simulink model "Final_Leg_PurePursuit_Squat_Climb"  (R2025b)
settings: Solver=ode45  StartTime=0.0  StopTime=150  MaxStep=0.002  RelTol=0.01  AbsTol=0.01  EnableMultiTasking=on
undefined symbols (not defined in the file): waypoints, X, Y, Z
libraries: sm_lib x81, nesl_utility x35, slpidlib x2, robotalgslib x1, sharedtransform x1
(part 4 of 5)

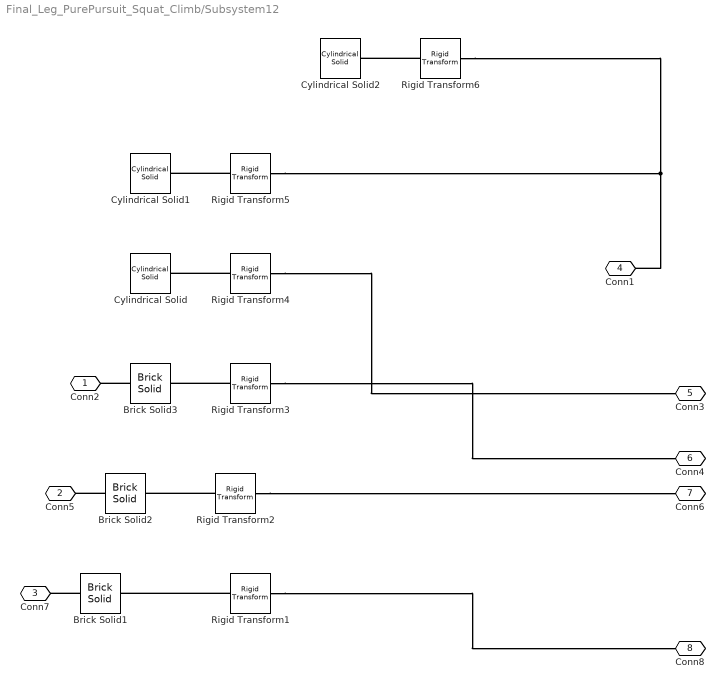
== system Final_Leg_PurePursuit_Squat_Climb/Subsystem12 ==
  Brick Solid1 : sm_lib/Body Elements/Brick Solid  BrickDimensions=[14.5 7.3 2]  BrickDimensionsUnits=m  ExportEntireGeometry=on  InertiaType=CalculateFromGeometry  BasedOnType=Density  Density=1000  DensityUnits=kg/m^3  Mass=1  MassUnits=kg  CenterOfMass=[0 0 0]  CenterOfMassUnits=m  MomentsOfInertia=[1 1 1]  MomentsOfInertiaUnits=kg*m^2  ProductsOfInertia=[0 0 0]  ProductsOfInertiaUnits=kg*m^2  GraphicType=FromGeometry  MarkerShape=Sphere  MarkerSize=10  GraphicVisPropType=SimpleVisualProperties  GraphicDiffuseColor=[0.3333 0.1882 0.007843]  GraphicOpacity=1  GraphicSpecularColor=[0.5 0.5 0.5 1.0]  GraphicAmbientColor=[0.15 0.15 0.15 1.0]  GraphicEmissiveColor=[0.0 0.0 0.0 1.0]  GraphicShininess=75  DoExposeReferenceFrame=on  SerializedFrames=<Frames/>
  Brick Solid2 : sm_lib/Body Elements/Brick Solid  BrickDimensions=[12.4 9.9 2]  BrickDimensionsUnits=m  ExportEntireGeometry=on  InertiaType=CalculateFromGeometry  BasedOnType=Density  Density=1000  DensityUnits=kg/m^3  Mass=1  MassUnits=kg  CenterOfMass=[0 0 0]  CenterOfMassUnits=m  MomentsOfInertia=[1 1 1]  MomentsOfInertiaUnits=kg*m^2  ProductsOfInertia=[0 0 0]  ProductsOfInertiaUnits=kg*m^2  GraphicType=FromGeometry  MarkerShape=Sphere  MarkerSize=10  GraphicVisPropType=SimpleVisualProperties  GraphicDiffuseColor=[0.3333 0.1882 0.007843]  GraphicOpacity=1  GraphicSpecularColor=[0.5 0.5 0.5 1.0]  GraphicAmbientColor=[0.15 0.15 0.15 1.0]  GraphicEmissiveColor=[0.0 0.0 0.0 1.0]  GraphicShininess=75  DoExposeReferenceFrame=on  SerializedFrames=<Frames/>
  Brick Solid3 : sm_lib/Body Elements/Brick Solid  BrickDimensions=[10 10 2]  BrickDimensionsUnits=m  ExportEntireGeometry=on  InertiaType=CalculateFromGeometry  BasedOnType=Density  Density=1000  DensityUnits=kg/m^3  Mass=1  MassUnits=kg  CenterOfMass=[0 0 0]  CenterOfMassUnits=m  MomentsOfInertia=[1 1 1]  MomentsOfInertiaUnits=kg*m^2  ProductsOfInertia=[0 0 0]  ProductsOfInertiaUnits=kg*m^2  GraphicType=FromGeometry  MarkerShape=Sphere  MarkerSize=10  GraphicVisPropType=SimpleVisualProperties  GraphicDiffuseColor=[0.3333 0.1882 0.007843]  GraphicOpacity=1  GraphicSpecularColor=[0.5 0.5 0.5 1.0]  GraphicAmbientColor=[0.15 0.15 0.15 1.0]  GraphicEmissiveColor=[0.0 0.0 0.0 1.0]  GraphicShininess=75  DoExposeReferenceFrame=on  SerializedFrames=<Frames/>
  Cylindrical Solid : sm_lib/Body Elements/Cylindrical Solid  CylinderRadius=6  CylinderRadiusUnits=m  CylinderLength=2  CylinderLengthUnits=m  ExportEntireGeometry=off  InertiaType=CalculateFromGeometry  BasedOnType=Density  Density=1000  DensityUnits=kg/m^3  Mass=1  MassUnits=kg  CenterOfMass=[0 0 0]  CenterOfMassUnits=m  MomentsOfInertia=[1 1 1]  MomentsOfInertiaUnits=kg*m^2  ProductsOfInertia=[0 0 0]  ProductsOfInertiaUnits=kg*m^2  GraphicType=FromGeometry  MarkerShape=Sphere  MarkerSize=10  GraphicVisPropType=SimpleVisualProperties  GraphicDiffuseColor=[0.3333 0.1882 0.007843]  GraphicOpacity=1  GraphicSpecularColor=[0.5 0.5 0.5 1.0]  GraphicAmbientColor=[0.15 0.15 0.15 1.0]  GraphicEmissiveColor=[0.0 0.0 0.0 1.0]  GraphicShininess=75  DoExposeReferenceFrame=on  SerializedFrames=<Frames/>
  Cylindrical Solid1 : sm_lib/Body Elements/Cylindrical Solid  CylinderRadius=5  CylinderRadiusUnits=m  CylinderLength=2  CylinderLengthUnits=m  ExportEntireGeometry=off  InertiaType=CalculateFromGeometry  BasedOnType=Density  Density=1000  DensityUnits=kg/m^3  Mass=1  MassUnits=kg  CenterOfMass=[0 0 0]  CenterOfMassUnits=m  MomentsOfInertia=[1 1 1]  MomentsOfInertiaUnits=kg*m^2  ProductsOfInertia=[0 0 0]  ProductsOfInertiaUnits=kg*m^2  GraphicType=FromGeometry  MarkerShape=Sphere  MarkerSize=10  GraphicVisPropType=SimpleVisualProperties  GraphicDiffuseColor=[0.3333 0.1882 0.007843]  GraphicOpacity=1  GraphicSpecularColor=[0.5 0.5 0.5 1.0]  GraphicAmbientColor=[0.15 0.15 0.15 1.0]  GraphicEmissiveColor=[0.0 0.0 0.0 1.0]  GraphicShininess=75  DoExposeReferenceFrame=on  SerializedFrames=<Frames/>
  Cylindrical Solid2 : sm_lib/Body Elements/Cylindrical Solid  CylinderRadius=5  CylinderRadiusUnits=m  CylinderLength=2  CylinderLengthUnits=m  ExportEntireGeometry=off  InertiaType=CalculateFromGeometry  BasedOnType=Density  Density=1000  DensityUnits=kg/m^3  Mass=1  MassUnits=kg  CenterOfMass=[0 0 0]  CenterOfMassUnits=m  MomentsOfInertia=[1 1 1]  MomentsOfInertiaUnits=kg*m^2  ProductsOfInertia=[0 0 0]  ProductsOfInertiaUnits=kg*m^2  GraphicType=FromGeometry  MarkerShape=Sphere  MarkerSize=10  GraphicVisPropType=SimpleVisualProperties  GraphicDiffuseColor=[0.3333 0.1882 0.007843]  GraphicOpacity=1  GraphicSpecularColor=[0.5 0.5 0.5 1.0]  GraphicAmbientColor=[0.15 0.15 0.15 1.0]  GraphicEmissiveColor=[0.0 0.0 0.0 1.0]  GraphicShininess=75  DoExposeReferenceFrame=on  SerializedFrames=<Frames/>
  Rigid Transform1 : sm_lib/Frames and Transforms/Rigid Transform  RotationMethod=None  FollAlignAxisA=+X  BaseAlignAxisA=+Y  FollAlignAxisB=+Y  BaseAlignAxisB=+Z  RotationStandardAxis=+Z  RotationAngle=90  RotationAngleUnits=deg  RotationArbitraryAxis=[0 0 1]  RotationSequenceAxes=FollowerAxes  RotationSequence=XYX  RotationSequenceAngles=[0 0 0]  RotationSequenceAnglesUnits=deg  RotationMatrix=[1 0 0;0 1 0;0 0 1]  Quaternion=[1 0 0 0]  TranslationMethod=Cartesian  TranslationCartesianOffset=[-15 -13.75 -1]  TranslationCartesianOffsetUnits=m  TranslationStandardAxis=+Z  TranslationStandardOffset=0  TranslationStandardOffsetUnits=m  TranslationROffset=0  TranslationROffsetUnits=m  TranslationThetaOffset=0  TranslationThetaOffsetUnits=deg  TranslationZOffset=0  TranslationZOffsetUnits=m
  Rigid Transform2 : sm_lib/Frames and Transforms/Rigid Transform  RotationMethod=None  FollAlignAxisA=+X  BaseAlignAxisA=+Y  FollAlignAxisB=+Y  BaseAlignAxisB=+Z  RotationStandardAxis=+Z  RotationAngle=90  RotationAngleUnits=deg  RotationArbitraryAxis=[0 0 1]  RotationSequenceAxes=FollowerAxes  RotationSequence=XYX  RotationSequenceAngles=[0 0 0]  RotationSequenceAnglesUnits=deg  RotationMatrix=[1 0 0;0 1 0;0 0 1]  Quaternion=[1 0 0 0]  TranslationMethod=Cartesian  TranslationCartesianOffset=[-21 -32.5 -1]  TranslationCartesianOffsetUnits=m  TranslationStandardAxis=+Z  TranslationStandardOffset=0  TranslationStandardOffsetUnits=m  TranslationROffset=0  TranslationROffsetUnits=m  TranslationThetaOffset=0  TranslationThetaOffsetUnits=deg  TranslationZOffset=0  TranslationZOffsetUnits=m
  Rigid Transform3 : sm_lib/Frames and Transforms/Rigid Transform  RotationMethod=None  FollAlignAxisA=+X  BaseAlignAxisA=+Y  FollAlignAxisB=+Y  BaseAlignAxisB=+Z  RotationStandardAxis=+Z  RotationAngle=90  RotationAngleUnits=deg  RotationArbitraryAxis=[0 0 1]  RotationSequenceAxes=FollowerAxes  RotationSequence=XYX  RotationSequenceAngles=[0 0 0]  RotationSequenceAnglesUnits=deg  RotationMatrix=[1 0 0;0 1 0;0 0 1]  Quaternion=[1 0 0 0]  TranslationMethod=Cartesian  TranslationCartesianOffset=[-37.5 -15 -1]  TranslationCartesianOffsetUnits=m  TranslationStandardAxis=+Z  TranslationStandardOffset=0  TranslationStandardOffsetUnits=m  TranslationROffset=0  TranslationROffsetUnits=m  TranslationThetaOffset=0  TranslationThetaOffsetUnits=deg  TranslationZOffset=0  TranslationZOffsetUnits=m
  Rigid Transform4 : sm_lib/Frames and Transforms/Rigid Transform  RotationMethod=None  FollAlignAxisA=+X  BaseAlignAxisA=+Y  FollAlignAxisB=+Y  BaseAlignAxisB=+Z  RotationStandardAxis=+Z  RotationAngle=90  RotationAngleUnits=deg  RotationArbitraryAxis=[0 0 1]  RotationSequenceAxes=FollowerAxes  RotationSequence=XYX  RotationSequenceAngles=[0 0 0]  RotationSequenceAnglesUnits=deg  RotationMatrix=[1 0 0;0 1 0;0 0 1]  Quaternion=[1 0 0 0]  TranslationMethod=Cartesian  TranslationCartesianOffset=[-15 -37.5 -1]  TranslationCartesianOffsetUnits=m  TranslationStandardAxis=+Z  TranslationStandardOffset=0  TranslationStandardOffsetUnits=m  TranslationROffset=0  TranslationROffsetUnits=m  TranslationThetaOffset=0  TranslationThetaOffsetUnits=deg  TranslationZOffset=0  TranslationZOffsetUnits=m
  Rigid Transform5 : sm_lib/Frames and Transforms/Rigid Transform  RotationMethod=None  FollAlignAxisA=+X  BaseAlignAxisA=+Y  FollAlignAxisB=+Y  BaseAlignAxisB=+Z  RotationStandardAxis=+Z  RotationAngle=90  RotationAngleUnits=deg  RotationArbitraryAxis=[0 0 1]  RotationSequenceAxes=FollowerAxes  RotationSequence=XYX  RotationSequenceAngles=[0 0 0]  RotationSequenceAnglesUnits=deg  RotationMatrix=[1 0 0;0 1 0;0 0 1]  Quaternion=[1 0 0 0]  TranslationMethod=Cartesian  TranslationCartesianOffset=[-35 -30 -1]  TranslationCartesianOffsetUnits=m  TranslationStandardAxis=+Z  TranslationStandardOffset=0  TranslationStandardOffsetUnits=m  TranslationROffset=0  TranslationROffsetUnits=m  TranslationThetaOffset=0  TranslationThetaOffsetUnits=deg  TranslationZOffset=0  TranslationZOffsetUnits=m
  Rigid Transform6 : sm_lib/Frames and Transforms/Rigid Transform  RotationMethod=None  FollAlignAxisA=+X  BaseAlignAxisA=+Y  FollAlignAxisB=+Y  BaseAlignAxisB=+Z  RotationStandardAxis=+Z  RotationAngle=90  RotationAngleUnits=deg  RotationArbitraryAxis=[0 0 1]  RotationSequenceAxes=FollowerAxes  RotationSequence=XYX  RotationSequenceAngles=[0 0 0]  RotationSequenceAnglesUnits=deg  RotationMatrix=[1 0 0;0 1 0;0 0 1]  Quaternion=[1 0 0 0]  TranslationMethod=Cartesian  TranslationCartesianOffset=[-25 -12.5 -1]  TranslationCartesianOffsetUnits=m  TranslationStandardAxis=+Z  TranslationStandardOffset=0  TranslationStandardOffsetUnits=m  TranslationROffset=0  TranslationROffsetUnits=m  TranslationThetaOffset=0  TranslationThetaOffsetUnits=deg  TranslationZOffset=0  TranslationZOffsetUnits=m
  Conn2 : PMIOPort  Side=Left
  Conn5 : PMIOPort  Port=2  Side=Left
  Conn7 : PMIOPort  Port=3  Side=Left
  Conn1 : PMIOPort  Port=4  Side=Right
  Conn3 : PMIOPort  Port=5  Side=Right
  Conn4 : PMIOPort  Port=6  Side=Right
  Conn6 : PMIOPort  Port=7  Side=Right
  Conn8 : PMIOPort  Port=8  Side=Right
  connections:
  Rigid Transform1/LConn1 -- Brick Solid1/RConn1
  Rigid Transform5/LConn1 -- Cylindrical Solid1/RConn1
  Rigid Transform3/LConn1 -- Brick Solid3/RConn1
  Rigid Transform5/RConn1 -- Conn1/RConn1 -- Rigid Transform6/RConn1
  Brick Solid2/LConn1 -- Conn5/RConn1
  Rigid Transform1/RConn1 -- Conn8/RConn1
  Rigid Transform4/RConn1 -- Conn3/RConn1
  Rigid Transform6/LConn1 -- Cylindrical Solid2/RConn1
  Rigid Transform4/LConn1 -- Cylindrical Solid/RConn1
  Rigid Transform2/LConn1 -- Brick Solid2/RConn1
  Rigid Transform3/RConn1 -- Conn4/RConn1
  Rigid Transform2/RConn1 -- Conn6/RConn1
  Brick Solid1/LConn1 -- Conn7/RConn1
  Brick Solid3/LConn1 -- Conn2/RConn1

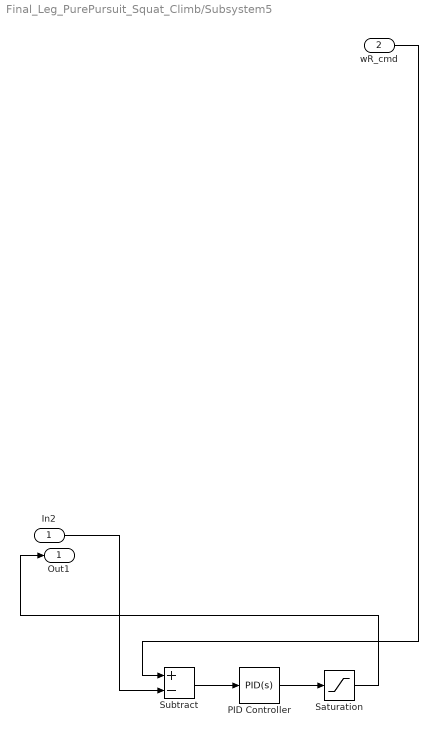
== system Final_Leg_PurePursuit_Squat_Climb/Subsystem5 ==
  In2 : Inport
  wR_cmd : Inport  Port=2
  PID Controller : slpidlib/PID Controller  Controller=PID  Form=Parallel  TimeDomain=Continuous-time  UseExternalTs=off  SampleTime=-1  IntegratorMethod=Forward Euler  FilterMethod=Forward Euler  ControllerParametersSource=internal  P=5  I=0  UseKiTs=off  D=0  UseExternalDerivativeSource=off  N=100  UseFilter=on  TunerSelectOption=Transfer Function Based (PID Tuner App)  InitialConditionSource=internal  InitialConditionForIntegrator=0  InitialConditionForFilter=0  DifferentiatorICPrevScaledInput=0  ExternalReset=none  TrackingMode=off  Kt=1  LimitOutput=off  SatLimitsSource=internal  UpperSaturationLimit=inf  LowerSaturationLimit=-inf  LinearizeAsGain=on  AntiWindupMode=none  Kb=1  LimitIntegrator=off  UpperIntegratorSaturationLimit=inf  LowerIntegratorSaturationLimit=-inf  POutMin=[]  POutMax=[]  IOutMin=[]  IOutMax=[]  DOutMin=[]  DOutMax=[]  NOutMin=[]  NOutMax=[]  SumOutMin=[]  SumOutMax=[]  SaturationOutMin=[]  SaturationOutMax=[]  PParamMin=[]  PParamMax=[]  IParamMin=[]  IParamMax=[]  DParamMin=[]  DParamMax=[]  NParamMin=[]  NParamMax=[]  KbParamMin=[]  KbParamMax=[]  KtParamMin=[]  KtParamMax=[]  KbOutMin=[]  KbOutMax=[]  KtOutMin=[]  KtOutMax=[]  IntegratorOutMin=[]  IntegratorOutMax=[]  FilterOutMin=[]  FilterOutMax=[]  SumI1OutMin=[]  SumI1OutMax=[]  SumI2OutMin=[]  SumI2OutMax=[]  SumI3OutMin=[]  SumI3OutMax=[]  SumI4OutMin=[]  SumI4OutMax=[]  SumDOutMin=[]  SumDOutMax=[]  DifferentiatorOutMin=[]  DifferentiatorOutMax=[]  FilterDiffOutCoefMin=[]  FilterDiffOutCoefMax=[]  ReciprocalOutMin=[]  ReciprocalOutMax=[]  SumDenOutMin=[]  SumDenOutMax=[]  SumNumOutMin=[]  SumNumOutMax=[]  DivideOutMin=[]  DivideOutMax=[]  UdiffTsProdOutMin=[]  UdiffTsProdOutMax=[]  NTsProdOutMin=[]  NTsProdOutMax=[]  UintegralTsProdOutMin=[]  UintegralTsProdOutMax=[]  UngainTsProdOutMin=[]  UngainTsProdOutMax=[]  ClampingZeroOutDataTypeStr=Inherit: Inherit via back propagation  ClampingZeroOutMin=[]  ClampingZeroOutMax=[]  FilterDenConstantOutDataTypeStr=Inherit: Inherit via back propagation  FilterDenConstantOutMin=[]  FilterDenConstantOutMax=[]  PCopyOutDataTypeStr=Inherit: Inherit via back propagation  PCopyOutMin=[]  PCopyOutMax=[]  NCopyOutDataTypeStr=Inherit: Inherit via back propagation  NCopyOutMin=[]  NCopyOutMax=[]  IntegratorContinuousStateAttributes=''  IntegratorStateMustResolveToSignalObject=off  IntegratorRTWStateStorageClass=Auto  FilterContinuousStateAttributes=''  FilterStateMustResolveToSignalObject=off  FilterRTWStateStorageClass=Auto  ParallelPVariant=InternalParameters  IdealPVariant=Disabled  IVariant=InternalParameters  DVariant=InternalParameters  IntegratorVariant=Continuous  SatVariant=Disabled  AWVariant=Passthrough  PCopyVariant=Disabled  TRVariant=Disabled  FdbkBlocksVariant=Forward  IdealPFdbkVariant=Disabled  SatFdbkVariant=Disabled  DerivativeFilterVariant=ContFilter  NVariant=InternalParameters  NCopyVariant=Disabled  FilterICVariant=InternalICsFilter  IntegratorICVariant=InternalICs  ExternalResetVariant=Disabled  TRSumVariant=Passthrough  SumFdbkVariant=Disabled  SumVariant=Sum_PID  TsampFilterVariant=InternalTs  TsampNgainVariant=Passthrough  TsampIntegralVariant=Disabled_SignalSpec  ExternalSaturationOutDataTypeStr=Inherit: Same as second input  DerivativeSourceVariant=ErrorSignal  PreIntVariant=InternalPreInt
  Saturation : Saturate  UpperLimit=5  LowerLimit=-5
  Subtract : Sum  Inputs=+-
  Out1 : Outport
  wires:
  In2/1 -> Subtract/2
  Subtract/1 -> PID Controller/1
  Saturation/1 -> Out1/1
  PID Controller/1 -> Saturation/1
  wR_cmd/1 -> Subtract/1

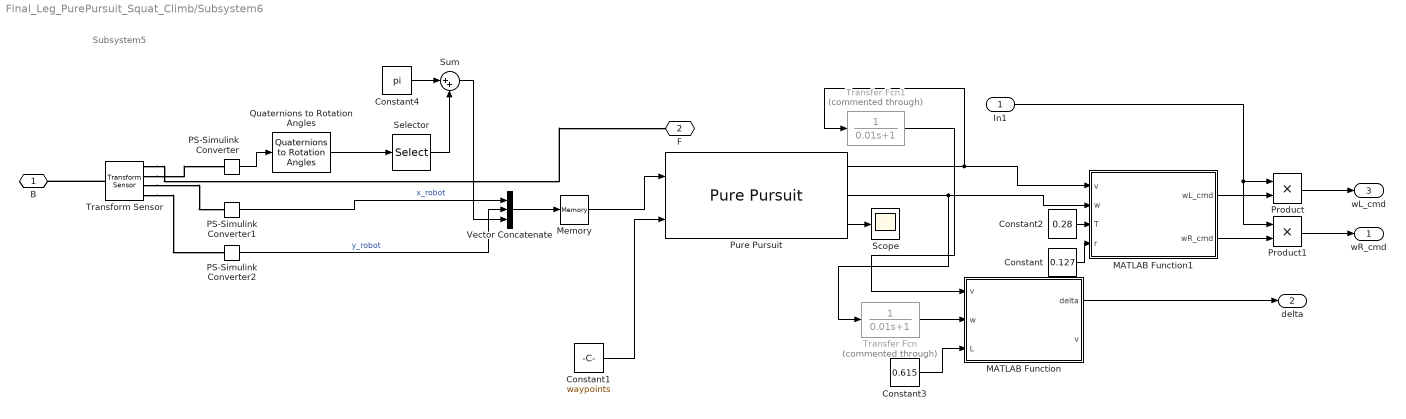
== system Final_Leg_PurePursuit_Squat_Climb/Subsystem6 ==
  note: Subsystem5
  In1 : Inport
  Constant : Constant  Value=0.127
  Constant1 : Constant  Value=waypoints
  Constant2 : Constant  Value=0.28
  Constant3 : Constant  Value=0.615
  Constant4 : Constant  Value=pi
  MATLAB Function : MATLAB Function  TreatAsAtomicUnit=on
  MATLAB Function1 : MATLAB Function  TreatAsAtomicUnit=on
  Memory : Memory
  PS-Simulink Converter : nesl_utility/PS-Simulink Converter  PhysicalDomain=network_engine_domain  SubClassName=ps_output  LeftPortType=input  RightPortType=output  PseudoPeriodic=off  Frequencies=[]  VectorFormat=inherit  Unit=inherit  AffineConversion=off
  PS-Simulink Converter1 : nesl_utility/PS-Simulink Converter  PhysicalDomain=network_engine_domain  SubClassName=ps_output  LeftPortType=input  RightPortType=output  PseudoPeriodic=off  Frequencies=[]  VectorFormat=inherit  Unit=inherit  AffineConversion=off
  PS-Simulink Converter2 : nesl_utility/PS-Simulink Converter  PhysicalDomain=network_engine_domain  SubClassName=ps_output  LeftPortType=input  RightPortType=output  PseudoPeriodic=off  Frequencies=[]  VectorFormat=inherit  Unit=inherit  AffineConversion=off
  Product : Product
  Product1 : Product
  Pure Pursuit : robotalgslib/Pure Pursuit  DesiredLinearVelocityPort=off  DesiredLinearVelocity=0.7  MaxAngularVelocity=0.8  LookaheadDistancePort=off  LookaheadDistance=0.6  TargetDirPort=on  SimulateUsing=Code generation
      settings: LibrarySourceBlock=navlib/Control Algorithms/Pure Pursuit
  Quaternions to Rotation Angles : sharedtransform/Quaternions to Rotation Angles  rotationOrder=ZYX  aMode=aMode
  Scope : Scope
      settings: ActiveDisplayYMinimum=-49.938512022124293  ActiveDisplayYMaximum=229.50278461957694
  Selector : Selector  InputPortWidth=3  IndexOptions=Index vector (dialog)  Indices=[1]  OutputSizes=1
  Sum : Sum  Inputs=|++
  Transfer Fcn : TransferFcn  Commented=through  Denominator=[0.01 1]
  Transfer Fcn1 : TransferFcn  Commented=through  Denominator=[0.01 1]
  Transform Sensor : sm_lib/Frames and Transforms/Transform Sensor  MeasurementFrame=World  RotationSequence=XYX  SenseAngle=off  SenseAxis=off  SenseQ=on  SenseR=off  SenseRotationSequence=off  SenseOmegaX=off  SenseOmegaY=off  SenseOmegaZ=off  SenseOmega=off  SenseQDot=off  SenseRDot=off  SenseRotationSequenceDot=off  SenseAlphaX=off  SenseAlphaY=off  SenseAlphaZ=off  SenseAlpha=off  SenseQDDot=off  SenseRDDot=off  SenseX=on  SenseY=on  SenseZ=off  SenseXYZ=off  SenseRad=off  SenseAzim=off  SenseDist=off  SenseInc=off  SenseXDot=off  SenseYDot=off  SenseZDot=off  SenseXYZDot=off  SenseRadDot=off  SenseAzimDot=off  SenseDistDot=off  SenseIncDot=off  SenseXDDot=off  SenseYDDot=off  SenseZDDot=off  SenseXYZDDot=off  SenseRadDDot=off  SenseAzimDDot=off  SenseDistDDot=off  SenseIncDDot=off
  Vector Concatenate : Concatenate  NumInputs=3
  B : PMIOPort  Side=Right
  F : PMIOPort  Port=2  Side=Right
  wR_cmd : Outport
  delta : Outport  Port=2
  wL_cmd : Outport  Port=3
  wires:
  Pure Pursuit/2 -> MATLAB Function1/2(w), Transfer Fcn/1
  Transfer Fcn1/1 -> MATLAB Function/1("v ")
  Transfer Fcn/1 -> MATLAB Function/2(w)
  Constant1/1 -> Pure Pursuit/2
  Constant/1 -> MATLAB Function1/4(r)
  Constant2/1 -> MATLAB Function1/3(T)
  Constant3/1 -> MATLAB Function/3(L)
  Pure Pursuit/1 -> MATLAB Function1/1(v), Transfer Fcn1/1
  Pure Pursuit/3 -> Scope/1
  Memory/1 -> Pure Pursuit/1
  In1/1 -> Product/1, Product1/1
  MATLAB Function1/1(wL_cmd) -> Product/2
  Product/1 -> wL_cmd/1
  MATLAB Function1/2(wR_cmd) -> Product1/2
  Product1/1 -> wR_cmd/1
  MATLAB Function/1(delta) -> delta/1
  Sum/1 -> Vector Concatenate/3
  Selector/1 -> Sum/2
  Constant4/1 -> Sum/1
  PS-Simulink Converter2/1 -> Vector Concatenate/2  "y_robot"
  PS-Simulink Converter1/1 -> Vector Concatenate/1  "x_robot"
  Vector Concatenate/1 -> Memory/1
  PS-Simulink Converter/1 -> Quaternions to Rotation Angles/1
  Quaternions to Rotation Angles/1 -> Selector/1
  connections:
  Transform Sensor/RConn1 -- F/RConn1
  Transform Sensor/LConn1 -- B/RConn1
  Transform Sensor/RConn3 -- PS-Simulink Converter1/LConn1
  Transform Sensor/RConn2 -- PS-Simulink Converter/LConn1
  Transform Sensor/RConn4 -- PS-Simulink Converter2/LConn1

== system Final_Leg_PurePursuit_Squat_Climb/Subsystem7 ==
  wL_cmd : Inport
  In2 : Inport  Port=2
  PID Controller : slpidlib/PID Controller  Controller=PID  Form=Parallel  TimeDomain=Continuous-time  UseExternalTs=off  SampleTime=-1  IntegratorMethod=Forward Euler  FilterMethod=Forward Euler  ControllerParametersSource=internal  P=5  I=0  UseKiTs=off  D=0  UseExternalDerivativeSource=off  N=100  UseFilter=on  TunerSelectOption=Transfer Function Based (PID Tuner App)  InitialConditionSource=internal  InitialConditionForIntegrator=0  InitialConditionForFilter=0  DifferentiatorICPrevScaledInput=0  ExternalReset=none  TrackingMode=off  Kt=1  LimitOutput=off  SatLimitsSource=internal  UpperSaturationLimit=inf  LowerSaturationLimit=-inf  LinearizeAsGain=on  AntiWindupMode=none  Kb=1  LimitIntegrator=off  UpperIntegratorSaturationLimit=inf  LowerIntegratorSaturationLimit=-inf  POutMin=[]  POutMax=[]  IOutMin=[]  IOutMax=[]  DOutMin=[]  DOutMax=[]  NOutMin=[]  NOutMax=[]  SumOutMin=[]  SumOutMax=[]  SaturationOutMin=[]  SaturationOutMax=[]  PParamMin=[]  PParamMax=[]  IParamMin=[]  IParamMax=[]  DParamMin=[]  DParamMax=[]  NParamMin=[]  NParamMax=[]  KbParamMin=[]  KbParamMax=[]  KtParamMin=[]  KtParamMax=[]  KbOutMin=[]  KbOutMax=[]  KtOutMin=[]  KtOutMax=[]  IntegratorOutMin=[]  IntegratorOutMax=[]  FilterOutMin=[]  FilterOutMax=[]  SumI1OutMin=[]  SumI1OutMax=[]  SumI2OutMin=[]  SumI2OutMax=[]  SumI3OutMin=[]  SumI3OutMax=[]  SumI4OutMin=[]  SumI4OutMax=[]  SumDOutMin=[]  SumDOutMax=[]  DifferentiatorOutMin=[]  DifferentiatorOutMax=[]  FilterDiffOutCoefMin=[]  FilterDiffOutCoefMax=[]  ReciprocalOutMin=[]  ReciprocalOutMax=[]  SumDenOutMin=[]  SumDenOutMax=[]  SumNumOutMin=[]  SumNumOutMax=[]  DivideOutMin=[]  DivideOutMax=[]  UdiffTsProdOutMin=[]  UdiffTsProdOutMax=[]  NTsProdOutMin=[]  NTsProdOutMax=[]  UintegralTsProdOutMin=[]  UintegralTsProdOutMax=[]  UngainTsProdOutMin=[]  UngainTsProdOutMax=[]  ClampingZeroOutDataTypeStr=Inherit: Inherit via back propagation  ClampingZeroOutMin=[]  ClampingZeroOutMax=[]  FilterDenConstantOutDataTypeStr=Inherit: Inherit via back propagation  FilterDenConstantOutMin=[]  FilterDenConstantOutMax=[]  PCopyOutDataTypeStr=Inherit: Inherit via back propagation  PCopyOutMin=[]  PCopyOutMax=[]  NCopyOutDataTypeStr=Inherit: Inherit via back propagation  NCopyOutMin=[]  NCopyOutMax=[]  IntegratorContinuousStateAttributes=''  IntegratorStateMustResolveToSignalObject=off  IntegratorRTWStateStorageClass=Auto  FilterContinuousStateAttributes=''  FilterStateMustResolveToSignalObject=off  FilterRTWStateStorageClass=Auto  ParallelPVariant=InternalParameters  IdealPVariant=Disabled  IVariant=InternalParameters  DVariant=InternalParameters  IntegratorVariant=Continuous  SatVariant=Disabled  AWVariant=Passthrough  PCopyVariant=Disabled  TRVariant=Disabled  FdbkBlocksVariant=Forward  IdealPFdbkVariant=Disabled  SatFdbkVariant=Disabled  DerivativeFilterVariant=ContFilter  NVariant=InternalParameters  NCopyVariant=Disabled  FilterICVariant=InternalICsFilter  IntegratorICVariant=InternalICs  ExternalResetVariant=Disabled  TRSumVariant=Passthrough  SumFdbkVariant=Disabled  SumVariant=Sum_PID  TsampFilterVariant=InternalTs  TsampNgainVariant=Passthrough  TsampIntegralVariant=Disabled_SignalSpec  ExternalSaturationOutDataTypeStr=Inherit: Same as second input  DerivativeSourceVariant=ErrorSignal  PreIntVariant=InternalPreInt
  Saturation : Saturate  UpperLimit=5  LowerLimit=-5
  Subtract : Sum  Inputs=+-
  Out1 : Outport
  wires:
  In2/1 -> Subtract/2
  Subtract/1 -> PID Controller/1
  Saturation/1 -> Out1/1
  PID Controller/1 -> Saturation/1
  wL_cmd/1 -> Subtract/1

== matlab function Final_Leg_PurePursuit_Squat_Climb/RL/MATLAB Function1 ==
  data: mode_cmd input; alpha input; tau output; q input; dq input; q_cmd input; is_locked output; q_ref output
function [tau, is_locked, q_ref] = LockJointPD(mode_cmd, alpha, q, dq, q_cmd)
%#codegen
% mode_cmd: 0=Walk (track q_cmd), 1=Wheeled (lock current angle)
% alpha   : [0,1] smoothing factor (TransferFcn output), 0=fully walking, 1=fully locked
% q,dq    : joint angle/angular velocity
% q_cmd   : walk/stand target angle (radians)
Kp = 1200.0;   % Starting value, tune per joint
Kd =   20.0;
tau_lim = 300.0;
m = uint8(mode_cmd ~= 0);     % Standardize to uint8(0/1)
a = double(alpha);
persistent q_hold last_mode
if isempty(q_hold),    q_hold    = q;        end   % double
if isempty(last_mode), last_mode = uint8(0); end   % uint8
% Rising edge: 0->1, latch current angle
if (last_mode == uint8(0)) && (m ~= uint8(0))
    q_hold = q;
end
last_mode = m;
% Reference angle: interpolate between "hold angle" and "target angle"
q_ref  = a*q_hold + (1-a)*q_cmd;
dq_ref = 0.0;
% PD
tau = Kp*(q_ref - q) + Kd*(dq_ref - dq);
% Saturation
tau = max(min(tau, tau_lim), -tau_lim);
% Debug flag: is leg lock dominant
is_locked = (a > 0.5);     % Can also output m==1
end

== matlab function Final_Leg_PurePursuit_Squat_Climb/Subsystem6/MATLAB Function1 ==
  data: v input; wL_cmd output; w input; T input; r input; wR_cmd output
function [wL_cmd, wR_cmd] = wheelSpeedCmd(v, w, T, r)
% v: linear velocity [m/s]
% w: yaw rate [rad/s]
% T: track width [m]
% r: wheel radius [m]

vL = v - 0.5*T*w;
vR = v + 0.5*T*w;

wL_cmd = vL / r;
wR_cmd = vR / r;
end

== matlab function Final_Leg_PurePursuit_Squat_Climb/Subsystem6/MATLAB Function ==
  data: v input; delta output; w input; L input; v output
function [delta, v] = Diff2Ackermann(v, w, L)
% input: 
%   v - Linear velocity (m/s)
%   w - Angular velocity (rad/s)
%   L - Wheelbase (m)
%
% output:
%   delta - front wheel rotation angel (rad)
%   v     -  velocity(m/s)
if abs(v) < 1e-3
    delta = 0;
else
    delta = atan(L * w / v);   % pure pursuit function
end

== matlab function Final_Leg_PurePursuit_Squat_Climb/RL/MATLAB Function3 ==
  data: brake_en input; tau output; w input
function tau = BrakeTorque(brake_en, w)
% brake_en: 0=brake disabled, 1= brake enabled
% w: Wheel angular velocity (rad/s)，output from Revolute Joint Velocity

Kb = 30.0;       % damping coefficient. Higher value=stronger braking
tau_max = 150.0; % maximal braking torque limit
w_eps = 0.05;    % velocity threshold to consider "stopped"

if brake_en == 0
    tau = 0.0;     % brake disabled
    return;
end

% stop applying torque at very low spped to prevent oscillation/jitter
if abs(w) < w_eps
    tau = 0.0;
else
    % damping braking: torque directtion is opposite to angular velocity
    tau = -Kb * w;
end

% torque saturation(limiting)
if tau >  tau_max, tau =  tau_max; end
if tau < -tau_max, tau = -tau_max; end
end

== matlab function Final_Leg_PurePursuit_Squat_Climb/RR/MATLAB Function2 ==
  data: t input; w output
function w = wheel_speed(t)
% ====================
% Parameter Definitions
% ====================
% --- Original Parameters ---
Tsw        = 105;   % Time to start initial acceleration
Tacc       = 2;     % Acceleration duration (0 -> V)
V          = 100;   % Target velocity magnitude 1 (Note: originally labeled as torque)
V2         = 20;    % Target velocity magnitude 2
Tdec_start = 125;   % Time to start deceleration (V -> 0)
Tdec       = 3;     % Deceleration duration
Tpause     = 5;     % Pause duration after stopping
Treacc     = 2;     % Re-acceleration duration (0 -> V2)

% --- New Parameters ---
Thold_V2   = 8;     % Duration to hold V2 (Code says 8s)
Tdec2      = 3;     % Second deceleration duration (V2 -> 0)
Tpause2    = 10;    % Second pause duration (Code says 10s)
Treacc2    = 2;     % Third acceleration duration (0 -> V2)

% ====================
% Time Node Calculation
% (Pre-calculating these improves readability and avoids errors)
% ====================
% Node 1: Time when first acceleration to V2 is complete (End of Phase 6)
T_V2_ready = Tdec_start + Tdec + Tpause + Treacc;

% Node 2: Time when holding V2 ends, start second deceleration
T_dec2_start = T_V2_ready + Thold_V2;

% Node 3: Time when second deceleration to 0 is complete
T_stop2_start = T_dec2_start + Tdec2;

% Node 4: Time when second pause ends, start final acceleration
T_last_acc_start = T_stop2_start + Tpause2;

% Node 5: Time when final acceleration to V2 is complete
T_final_stable = T_last_acc_start + Treacc2;

% ====================
% Logic Control
% ====================
% Phase 1: Not started (Idle)
if t < Tsw
    w = 0;

% Phase 2: Linear Acceleration 0 -> V
elseif t < Tsw + Tacc
    u = (t - Tsw) / Tacc;
    w = u * V;

% Phase 3: Hold V (Constant speed)
elseif t < Tdec_start
    w = V;

% Phase 4: Linear Deceleration V -> 0
elseif t < Tdec_start + Tdec
    u = (t - Tdec_start) / Tdec;
    w = V * (1 - u);

% Phase 5: Stop and Wait (Pause 1)
elseif t < Tdec_start + Tdec + Tpause
    w = 0;

% Phase 6: Re-accelerate 0 -> V2
elseif t < T_V2_ready
    u = (t - (Tdec_start + Tdec + Tpause)) / Treacc;
    w = u * V2;

% --------------------
% New Phases
% --------------------
% Phase 7: Hold V2
elseif t < T_dec2_start
    w = V2;

% Phase 8: Second Deceleration V2 -> 0
elseif t < T_stop2_start
    u = (t - T_dec2_start) / Tdec2;
    w = V2 * (1 - u);

% Phase 9: Second Stop and Wait (Pause 2)
elseif t < T_last_acc_start
    w = 0;

% Phase 10: Final Acceleration 0 -> V2
elseif t < T_final_stable
    u = (t - T_last_acc_start) / Treacc2;
    w = u * V2;

% Phase 11: Hold V2 indefinitely
else
    w = V2;
end
end

== matlab function Final_Leg_PurePursuit_Squat_Climb/Front_left_gait/MATLAB Function2 ==
  data: t input; q output; mode_cmd input
function q = hip_FL_motion(t, mode_cmd)
% --- Front Left (FL) Hip Joint Motion Planner ---

% ====================
% Time Node Definitions
% ====================
T_squat_start = 102;  % Squat start time
T_climb_start = 130;  % Climb start time

% ====================
% Phase 0: Wheeled Mode or Not Started
% ====================
if (mode_cmd == 1) || (t < T_squat_start)
    q = 0; 
    return;
end

% ==========================================
% Phase 1: Static Squat Test (102s ~ 130s)
% ==========================================
if t < T_climb_start
    tau = t - T_squat_start; % Local time / Elapsed time
    
    % Squat Parameters
    q_stand = 0;
    q_squat = deg2rad(35);   % Squat angle
    T1 = 3; T2 = 15; T3 = 3; % Action durations
    
    if tau < T1
        u = tau / T1;
        q = (1-u)*q_stand + u*q_squat;
    elseif tau < T1 + T2
        q = q_squat;
    elseif tau < T1 + T2 + T3
        u = (tau - (T1 + T2)) / T3;
        q = (1-u)*q_squat + u*q_stand;
    else
        q = q_stand; % 123s~130s: Hold standing position and wait
    end
    return;
end

% ==========================================
% Phase 2: Stair Climbing Motion (Starts at 130s)
% ==========================================
% Reset local time, counting from 130s
tau = t - T_climb_start; 

% Climbing Parameters
q_stand = 0;
q_lift  = deg2rad(-30);  % [Lift] Negative value to lift up and clear the step
q_step  = deg2rad(20);   % [Landing] Positive value to land on step, adapting to height diff

% Time Allocation
T_up   = 2.0;   % Duration to lift
T_hold = 9.0;   % Hold in air (Allow time for rear wheels to drive forward)
T_down = 2.0;   % Duration to lower

if tau < T_up
    % 1. Lift Leg (Swing Up)
    u = tau / T_up;
    q = (1-u)*q_stand + u*q_lift;
    
elseif tau < (T_up + T_hold)
    % 2. Maintain Height (Vehicle should move forward now)
    q = q_lift;
    
elseif tau < (T_up + T_hold + T_down)
    % 3. Lower Leg (Land on the step)
    dt = tau - (T_up + T_hold);
    u = dt / T_down;
    q = (1-u)*q_lift + u*q_step;
    
else
    % 4. Maintain Stance on Step
    % (Keep this pose until all legs are up, then reset to 0 together)
    q = q_step;
end
end

== matlab function Final_Leg_PurePursuit_Squat_Climb/Front_left_gait/MATLAB Function3 ==
  data: t input; q output; mode_cmd input
function q = knee_FL_motion(t, mode_cmd)
% --- Front Left (FL) Knee Joint Motion Planner ---

% ====================
% Time Node Definitions
% ====================
T_squat_start = 102;
T_climb_start = 130;

% ====================
% Phase 0: Wheeled Mode (Idle)
% ====================
if (mode_cmd == 1) || (t < T_squat_start)
    q = 0;
    return;
end

% ==========================================
% Phase 1: Static Squat Test (102s ~ 130s)
% ==========================================
if t < T_climb_start
    tau = t - T_squat_start;
    
    % Squat Parameters
    q_stand = 0;
    q_squat = -deg2rad(70);  % Squat angle
    T1 = 3;   % Descent time
    T2 = 15;  % Hold time
    T3 = 3;   % Ascent time
    
    if tau < T1
        u = tau / T1;
        q = (1-u)*q_stand + u*q_squat;
    elseif tau < T1 + T2
        q = q_squat;
    elseif tau < T1 + T2 + T3
        u = (tau - (T1 + T2)) / T3;
        q = (1-u)*q_squat + u*q_stand;
    else
        q = q_stand;
    end
    return;
end

% ==========================================
% Phase 2: Stair Climbing Motion (Starts at 130s)
% ==========================================
tau = t - T_climb_start;

% Climbing Parameters
q_stand = 0;
q_lift  = deg2rad(-30);  % [Critical] Large knee bend to retract/lift the wheel
q_step  = deg2rad(-90);  % [Landing] Land on step, slight bend for damping/buffering

% Motion Timing Distribution (Must match Hip strictly)
T_up   = 2.0;
T_hold = 9.0;
T_down = 2.0;

if tau < T_up
    % 1. Lift Leg (Retraction)
    u = tau / T_up;
    q = (1-u)*q_stand + u*q_lift;
    
elseif tau < (T_up + T_hold)
    % 2. Hold High
    q = q_lift;
    
elseif tau < (T_up + T_hold + T_down)
    % 3. Lower Leg (Placement)
    dt = tau - (T_up + T_hold);
    u = dt / T_down;
    q = (1-u)*q_lift + u*q_step;
    
else
    % 4. Maintain stance on the step
    q = q_step;
end
end

== matlab function Final_Leg_PurePursuit_Squat_Climb/RR/MATLAB Function1 ==
  data: mode_cmd input; alpha input; tau output; q input; dq input; q_cmd input; is_locked output; q_ref output
function [tau, is_locked, q_ref] = LockJointPD(mode_cmd, alpha, q, dq, q_cmd)
%#codegen
% mode_cmd: 0=Walk (track q_cmd), 1=Wheeled (lock current angle)
% alpha   : [0,1] smoothing factor (TransferFcn output), 0=fully walking, 1=fully locked
% q,dq    : joint angle/angular velocity
% q_cmd   : walk/stand target angle (radians)
Kp = 1200.0;   % Starting value, tune per joint
Kd =   20.0;
tau_lim = 300.0;
m = uint8(mode_cmd ~= 0);     % Standardize to uint8(0/1)
a = double(alpha);
persistent q_hold last_mode
if isempty(q_hold),    q_hold    = q;        end   % double
if isempty(last_mode), last_mode = uint8(0); end   % uint8
% Rising edge: 0->1, latch current angle
if (last_mode == uint8(0)) && (m ~= uint8(0))
    q_hold = q;
end
last_mode = m;
% Reference angle: interpolate between "hold angle" and "target angle"
q_ref  = a*q_hold + (1-a)*q_cmd;
dq_ref = 0.0;
% PD
tau = Kp*(q_ref - q) + Kd*(dq_ref - dq);
% Saturation
tau = max(min(tau, tau_lim), -tau_lim);
% Debug flag: is leg lock dominant
is_locked = (a > 0.5);     % Can also output m==1
end

== matlab function Final_Leg_PurePursuit_Squat_Climb/RR/MATLAB Function3 ==
  data: brake_en input; tau output; w input
function tau = BrakeTorque(brake_en, w)
% brake_en: 0=brake disabled, 1= brake enabled
% w: Wheel angular velocity (rad/s)，output from Revolute Joint Velocity

Kb = 30.0;       % damping coefficient. Higher value=stronger braking
tau_max = 150.0; % maximal braking torque limit
w_eps = 0.05;    % velocity threshold to consider "stopped"

if brake_en == 0
    tau = 0.0;     % brake disabled
    return;
end

% stop applying torque at very low spped to prevent oscillation/jitter
if abs(w) < w_eps
    tau = 0.0;
else
    % damping braking: torque directtion is opposite to angular velocity
    tau = -Kb * w;
end

% torque saturation(limiting)
if tau >  tau_max, tau =  tau_max; end
if tau < -tau_max, tau = -tau_max; end
end

== matlab function Final_Leg_PurePursuit_Squat_Climb/Front_right_gait/MATLAB Function1 ==
  data: t input; q output; mode_cmd input
function q = hip_FR_motion(t, mode_cmd)
% --- Front Right (FR) Hip Joint Motion Planner ---

% ====================
% Time Node Definitions
% ====================
T_squat_start = 102;  % Squat start time
T_climb_start = 135;  % Climb start time (Updated to 135s)

% ====================
% Phase 0: Wheeled Mode or Not Started
% ====================
if (mode_cmd == 1) || (t < T_squat_start)
    q = 0; 
    return;
end

% ==========================================
% Phase 1: Static Squat Test (102s ~ 135s)
% ==========================================
if t < T_climb_start
    tau = t - T_squat_start; % Local time / Elapsed time
    
    % Squat Parameters
    q_stand = 0;
    q_squat = deg2rad(35);   % Squat angle
    T1 = 3; T2 = 15; T3 = 3; % Action durations
    
    if tau < T1
        u = tau / T1;
        q = (1-u)*q_stand + u*q_squat;
    elseif tau < T1 + T2
        q = q_squat;
    elseif tau < T1 + T2 + T3
        u = (tau - (T1 + T2)) / T3;
        q = (1-u)*q_squat + u*q_stand;
    else
        q = q_stand; % 123s~135s: Hold standing position and wait
    end
    return;
end

% ==========================================
% Phase 2: Stair Climbing Motion (Starts at 135s)
% ==========================================
% Reset local time, counting from 135s
tau = t - T_climb_start; 

% Climbing Parameters
q_stand = 0;
q_lift  = deg2rad(-30);  % [Lift] Negative value to lift up and clear the step
q_step  = deg2rad(20);   % [Landing] Land on step, keep slightly bent to adapt to height diff

% Time Allocation
T_up   = 2.0;   % Duration to lift
T_hold = 4.0;   % Hold in air (Allow time for rear wheels to drive forward)
T_down = 2.0;   % Duration to lower

if tau < T_up
    % 1. Lift Leg (Swing Up)
    u = tau / T_up;
    q = (1-u)*q_stand + u*q_lift;
    
elseif tau < (T_up + T_hold)
    % 2. Maintain Height (Vehicle should move forward now)
    q = q_lift;
    
elseif tau < (T_up + T_hold + T_down)
    % 3. Lower Leg (Land on the step)
    dt = tau - (T_up + T_hold);
    u = dt / T_down;
    q = (1-u)*q_lift + u*q_step;
    
else
    % 4. Maintain Stance on Step
    % (Keep this pose until all legs are up, then reset to 0 together)
    q = q_step;
end
end

== matlab function Final_Leg_PurePursuit_Squat_Climb/Front_right_gait/MATLAB Function4 ==
  data: t input; q output; mode_cmd input
function q = knee_FR_motion(t, mode_cmd)
% --- Front Left (FL) Knee Joint Motion Planner ---

% ====================
% Time Node Definitions
% ====================
T_squat_start = 102;
T_climb_start = 135;  % [Updated] Climb start time moved to 135s

% ====================
% Phase 0: Wheeled Mode (Idle)
% ====================
if (mode_cmd == 1) || (t < T_squat_start)
    q = 0;
    return;
end

% ==========================================
% Phase 1: Static Squat Test (102s ~ 135s)
% ==========================================
if t < T_climb_start
    tau = t - T_squat_start;
    
    % Squat Parameters
    q_stand = 0;
    q_squat = -deg2rad(70);  % Squat angle
    T1 = 3;   % Descent time
    T2 = 15;  % Hold time
    T3 = 3;   % Ascent time
    
    if tau < T1
        u = tau / T1;
        q = (1-u)*q_stand + u*q_squat;
    elseif tau < T1 + T2
        q = q_squat;
    elseif tau < T1 + T2 + T3
        u = (tau - (T1 + T2)) / T3;
        q = (1-u)*q_squat + u*q_stand;
    else
        q = q_stand;
    end
    return;
end

% ==========================================
% Phase 2: Stair Climbing Motion (Starts at 135s)
% ==========================================
tau = t - T_climb_start;

% Climbing Parameters
q_stand = 0;
q_lift  = deg2rad(-30);  % [Critical] Large knee bend to retract/lift the wheel
q_step  = deg2rad(-90);  % [Landing] Land on step, slight bend for damping/buffering

% Motion Timing Distribution (Must match Hip strictly)
T_up   = 2.0;
T_hold = 4.0;    % [Updated] Hold time reduced to 4s
T_down = 2.0;

if tau < T_up
    % 1. Lift Leg (Retraction)
    u = tau / T_up;
    q = (1-u)*q_stand + u*q_lift;
    
elseif tau < (T_up + T_hold)
    % 2. Hold High
    q = q_lift;
    
elseif tau < (T_up + T_hold + T_down)
    % 3. Lower Leg (Placement)
    dt = tau - (T_up + T_hold);
    u = dt / T_down;
    q = (1-u)*q_lift + u*q_step;
    
else
    % 4. Maintain stance on the step
    q = q_step;
end
end

== matlab function Final_Leg_PurePursuit_Squat_Climb/Rear_right_gait/MATLAB Function2 ==
  data: t input; q output; mode_cmd input
function q = hip_RL_motion(t, mode_cmd)
% --- Rear Left (RL) Hip Joint Motion Planner ---

% ====================
% Time Node Definitions
% ====================
T_squat_start = 102;
T_tuck_start  = 146;  % Tuck preparation start time
T_climb_start = 160;  % Climb start time (Synced with Knee)

% ====================
% Phase 0: Wheeled Mode (Idle)
% ====================
if (mode_cmd == 1) || (t < T_squat_start)
    q = 0; 
    return;
end

% ==========================================
% Phase 1: Static Squat Test (102s ~ 146s)
% ==========================================
if t < T_tuck_start
    tau = t - T_squat_start;
    q_stand = 0;
    q_squat = deg2rad(35);   % Squat angle (Positive)
    T1 = 3; T2 = 15; T3 = 3;
    
    if tau < T1
        u = tau / T1;
        q = (1-u)*q_stand + u*q_squat;
    elseif tau < T1 + T2
        q = q_squat;
    elseif tau < T1 + T2 + T3
        u = (tau - (T1 + T2)) / T3;
        q = (1-u)*q_squat + u*q_stand;
    else
        q = q_stand;
    end
    return;
end

% ==========================================
% Phase 2: Tuck Preparation (146s ~ 160s)
% ==========================================
% The hip joint usually stays near 0 or applies a slight angle to coordinate
% with the knee retraction.
q_stand = 0;
q_tuck  = deg2rad(5); % Slight positive angle to assist tucking
if t < T_climb_start
    tau = t - T_tuck_start;
    T_transition = 5.0;
    
    if tau < T_transition
        u = tau / T_transition;
        q = (1-u)*q_stand + u*q_tuck;
    else
        % Hold tuck position
        q = q_tuck;
    end
    return;
end

% ==========================================
% Phase 3: Stair Climbing Motion (Starts at 160s)
% ==========================================
tau = t - T_climb_start;

% Climbing Parameters
q_lift  = deg2rad(-25);  % [Lift] Swing leg up
q_step  = deg2rad(-10);  % [Landing] Stance on step
T_up   = 2.0;
T_hold = 3.0;
T_down = 2.0;

if tau < T_up
    % 1. Transition: Tuck -> Lift
    % (Starting from q_tuck ensures smooth motion)
    u = tau / T_up;
    q = (1-u)*q_tuck + u*q_lift;
    
elseif tau < (T_up + T_hold)
    % 2. Hold High
    q = q_lift;
    
elseif tau < (T_up + T_hold + T_down)
    % 3. Lower Leg (Landing)
    dt = tau - (T_up + T_hold);
    u = dt / T_down;
    q = (1-u)*q_lift + u*q_step;
    
else
    % 4. Maintain Stance on Step
    q = q_step;
end
end

== matlab function Final_Leg_PurePursuit_Squat_Climb/Rear_right_gait/MATLAB Function3 ==
  data: t input; q output; mode_cmd input
function q = knee_RL_motion(t, mode_cmd)
% --- Rear Left (RL) Knee Joint Motion Planner ---

% ====================
% Time Node Definitions
% ====================
T_squat_start = 102;
T_tuck_start  = 146;  % [New] Time to start tucking legs (Preparation after front legs are done)
T_climb_start = 160;  % [Updated] Time to start actual stair climbing motion

% ====================
% Phase 0: Wheeled Mode (Idle)
% ====================
if (mode_cmd == 1) || (t < T_squat_start)
    q = 0; 
    return;
end

% ==========================================
% Phase 1: Static Squat Test (102s ~ 146s)
% ==========================================
if t < T_tuck_start
    tau = t - T_squat_start;
    q_stand = 0;
    q_squat = -deg2rad(70);
    T1 = 3; T2 = 15; T3 = 3;
    
    if tau < T1
        u = tau / T1;
        q = (1-u)*q_stand + u*q_squat;
    elseif tau < T1 + T2
        q = q_squat;
    elseif tau < T1 + T2 + T3
        u = (tau - (T1 + T2)) / T3;
        q = (1-u)*q_squat + u*q_stand;
    else
        q = q_stand;
    end
    return;
end

% ==========================================
% Phase 2: [New] Tuck Preparation (146s ~ 160s)
% Core Strategy: Retract rear wheels forward to shorten the lever arm
% and prevent tipping over (anti-tipping logic).
% ==========================================
q_stand = 0;
q_tuck  = deg2rad(-20);  % Tuck angle: Bend knee to pull wheels in (Retract)

if t < T_climb_start
    tau = t - T_tuck_start;
    T_transition = 5.0; % Retract slowly over 5 seconds
    
    if tau < T_transition
        u = tau / T_transition;
        q = (1-u)*q_stand + u*q_tuck;
    else
        % Hold the tucked position, waiting for climb signal
        q = q_tuck; 
    end
    return;
end

% ==========================================
% Phase 3: Stair Climbing Motion (Starts at 160s)
% ==========================================
tau = t - T_climb_start;

% Climbing Parameters
% NOTE: The starting point is now 'q_tuck', not 'q_stand'
q_lift  = deg2rad(-80);  % [Important] High lift: Bend deep to clear the step
q_step  = deg2rad(-20);  % [Landing] Land on step, slight bend
T_up   = 2.0;
T_hold = 3.0;
T_down = 2.0;

if tau < T_up
    % 1. Transition: Tuck -> Lift
    u = tau / T_up;
    q = (1-u)*q_tuck + u*q_lift; % Interpolate from Tuck angle
    
elseif tau < (T_up + T_hold)
    % 2. Hold High
    q = q_lift;
    
elseif tau < (T_up + T_hold + T_down)
    % 3. Lower Leg (Landing)
    dt = tau - (T_up + T_hold);
    u = dt / T_down;
    q = (1-u)*q_lift + u*q_step;
    
else
    % 4. Maintain stance on the step
    q = q_step;
end
end

== matlab function Final_Leg_PurePursuit_Squat_Climb/Rear_left_gait/MATLAB Function2 ==
  data: t input; q output; mode_cmd input
function q = hip_RL_motion(t, mode_cmd)
% --- Rear Left (RL) Hip Joint Motion Planner ---

% ====================
% Time Nodes
% ====================
T_squat_start = 102;
T_tuck_start  = 146;
T_climb_start = 155;

% ====================
% Phase 0: Wheeled Mode (Idle)
% ====================
if (mode_cmd == 1) || (t < T_squat_start)
    q = 0; 
    return;
end

% ==========================================
% Phase 1: Static Squat Test (102s ~ 130s)
% ==========================================
if t < T_tuck_start
    tau = t - T_squat_start;
    q_stand = 0;
    q_squat = deg2rad(35); % Positive angle for squatting (adjust based on coord system)
    T1 = 3;   % Descent time
    T2 = 15;  % Hold time
    T3 = 3;   % Ascent time
    
    if tau < T1
        u = tau / T1;
        q = (1-u)*q_stand + u*q_squat;
    elseif tau < T1 + T2
        q = q_squat;
    elseif tau < T1 + T2 + T3
        u = (tau - (T1 + T2)) / T3;
        q = (1-u)*q_squat + u*q_stand;
    else
        q = q_stand;
    end
    return;
end

% ==========================================
% Phase 2: Tuck Preparation (130s ~ 153s)
% ==========================================
% The hip joint usually stays at 0 during tuck, or applies a slight angle to coordinate.
q_stand = 0;
q_tuck  = deg2rad(5); % Apply a slight positive angle (or 0), depending on the situation
if t < T_climb_start
    tau = t - T_tuck_start;
    T_transition = 5.0;
    
    if tau < T_transition
        u = tau / T_transition;
        q = (1-u)*q_stand + u*q_tuck;
    else
        q = q_tuck;
    end
    return;
end

% ==========================================
% Phase 3: Stair Climbing Motion (Starts at 153s)
% ==========================================
tau = t - T_climb_start;

% Climbing Parameters
q_lift  = deg2rad(-25);  % Lift leg (Swing phase)
q_step  = deg2rad(-10);  % Landing on step (Stance phase)
T_up   = 2.0;            % Time to lift
T_hold = 3.0;            % Time to hold
T_down = 2.0;            % Time to lower

if tau < T_up
    % Transition: Lift starting from q_tuck
    u = tau / T_up;
    q = (1-u)*q_tuck + u*q_lift;
    
elseif tau < (T_up + T_hold)
    q = q_lift;
    
elseif tau < (T_up + T_hold + T_down)
    dt = tau - (T_up + T_hold);
    u = dt / T_down;
    q = (1-u)*q_lift + u*q_step;
    
else
    q = q_step;
end
end

== matlab function Final_Leg_PurePursuit_Squat_Climb/Rear_left_gait/MATLAB Function4 ==
  data: t input; q output; mode_cmd input
function q = knee_RL_motion(t, mode_cmd)
% --- Rear Left (RL) Knee Joint Motion Planner ---

% ====================
% Time Nodes
% ====================
T_squat_start = 102;
T_tuck_start  = 146;  % [New] Time to start tucking legs (Preparation)
T_climb_start = 155;  % Time to start actual stair climbing

% ====================
% Phase 0: Wheeled Mode (Idle)
% ====================
if (mode_cmd == 1) || (t < T_squat_start)
    q = 0; 
    return;
end

% ==========================================
% Phase 1: Static Squat Test (102s ~ 130s)
% ==========================================
if t < T_tuck_start
    tau = t - T_squat_start;
    q_stand = 0;
    q_squat = -deg2rad(70);
    T1 = 3;   % Descent time
    T2 = 15;  % Hold time
    T3 = 3;   % Ascent time
    
    if tau < T1
        u = tau / T1;
        q = (1-u)*q_stand + u*q_squat;
    elseif tau < T1 + T2
        q = q_squat;
    elseif tau < T1 + T2 + T3
        u = (tau - (T1 + T2)) / T3;
        q = (1-u)*q_squat + u*q_stand;
    else
        q = q_stand;
    end
    return;
end

% ==========================================
% Phase 2: [New] Tuck Preparation (130s ~ 153s)
% Core Strategy: Retract rear wheels forward to shorten the lever arm
% and prevent tipping over during the wait.
% ==========================================
q_stand = 0;
q_tuck  = deg2rad(-20);  % Tuck angle: Bend knee 20 deg to pull wheels in

if t < T_climb_start
    tau = t - T_tuck_start;
    T_transition = 5.0; % Retract slowly over 5 seconds
    
    if tau < T_transition
        u = tau / T_transition;
        q = (1-u)*q_stand + u*q_tuck;
    else
        % Hold the tucked position, waiting for jump/climb signal
        q = q_tuck; 
    end
    return;
end

% ==========================================
% Phase 3: Stair Climbing Motion (Starts at 153s)
% ==========================================
tau = t - T_climb_start;

% Climbing Parameters
% NOTE: The starting point is now 'q_tuck', not 'q_stand'
q_lift  = deg2rad(-80);  % [Important] High lift: Bend deep to clear the step
q_step  = deg2rad(-20);  % Landing: Slightly bent after mounting step
T_up   = 2.0;            % Time to lift
T_hold = 3.0;            % Time to hold in air
T_down = 2.0;            % Time to lower leg

if tau < T_up
    % 1. Transition: Tuck -> Lift
    u = tau / T_up;
    q = (1-u)*q_tuck + u*q_lift; % Interpolate from Tuck angle
    
elseif tau < (T_up + T_hold)
    % 2. Hold High
    q = q_lift;
    
elseif tau < (T_up + T_hold + T_down)
    % 3. Lower Leg (Landing)
    dt = tau - (T_up + T_hold);
    u = dt / T_down;
    q = (1-u)*q_lift + u*q_step;
    
else
    % 4. Stay on Step
    q = q_step;
end
end
